simulink library "ModelsLibrary"  (R2017b)
settings: Solver=VariableStepAuto  StartTime=0.0  StopTime=10.0  RelTol=1e-3
libraries: sharedutil x3, simulink x2, ModelsLibrary x2
settings Model: Creator=AHKh  LastModifiedBy=AHKh
settings CodeAppCC: StateflowObjectComments=on

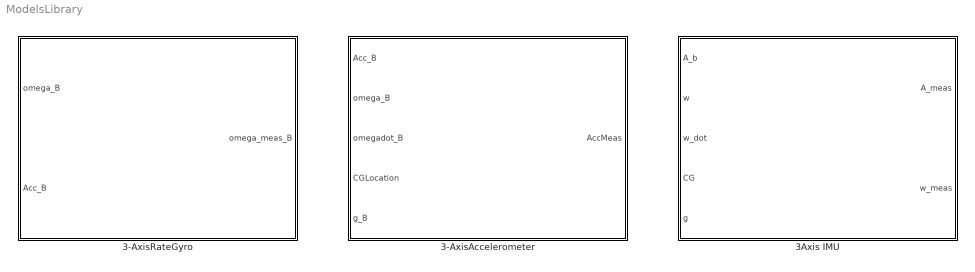
== system ModelsLibrary ==
  3-AxisAccelerometer : Subsystem  mask{units=Metric (MKS), SensorLoc=[0; 0; 0], gtype=off, dtype_a=on, w_a=190, z_a=0.707, SFCC=eye(3), SensorBias=[0; 0; 0], Ts=0.001, AccNoiseCheck=on, NoiseSeeds=[23093; 23094; 23095], NoisePower=[0.001; 0.001; 0.001], satUpper=[inf; inf; inf], satLower=[-inf; -inf; -inf]}
      mask prompts: units "Unit"; SensorLoc "Accelerometer Location"; gtype "Subtracting Gravity"; dtype_a "Considering 2nd-Order Dynamics"; w_a "Natural Frequency (rad/s)"; z_a "Damping Ratio"; SFCC "Scale Factor and Cross-Coupling"; SensorBias "Measurment Bias"; Ts "Update Rate (sec)"; AccNoiseCheck "Considering Noise"; NoiseSeeds "Noise Seeds"; NoisePower "Noise Power"; satUpper "Output Upper Limits"; satLower "Output Lower Limits"
      mask TypeOptions units: Metric (MKS)
      mask DialogControl DescGroupVar Prompt: Three-Axis Accelerometer
      mask DialogControl DescTextVar Prompt: Implements a three-axis accelerometer
      mask DialogControl Container4 Prompt: Main
      mask DialogControl units Tooltip: Metric System of Units
      mask DialogControl Container5 Prompt: Noise Characteristics
      mask Display:
      | port_label('input',1,'[Acc]^{B}_B (m/s^2)','texmode','on');
      | port_label('input',2,'[\omega]^B_B (rad/s)','texmode','on');
      | port_label('input',3,'[d\omega/dt]^B_B (rad/s^2)','texmode','on');
      | port_label('input',4,'[CG]^B_B (m)','texmode','on');
      | port_label('input',5,'[g]^B_B (m/s^2)','texmode','on');
      | port_label('output',1,'[Acc_{meas}]^{B}_B (m/s^2)','texmode','on');
  3-AxisRateGyro : Subsystem  mask(Three-Axis Rate Gyroscope){dtype_g=on, w_g=190, z_g=0.707, SFCC=eye(3), SensorBias=[0; 0; 0], gSensitivity=[0; 0; 0], Ts=0.001, GyroNoiseCheck=on, NoiseSeeds=[23093; 23094; 23095], NoisePower=[0.0001; 0.0001; 0.0001], satUpper=[inf; inf; inf], satLower=[-inf; -inf; -inf]}
      mask prompts: dtype_g "Considering 2nd-Order Dynamics"; w_g "Natural Frequency (rad/s)"; z_g "Damping Ratio"; SFCC "Scale Factors and Cross-Coupling"; SensorBias "Measurment Bias"; gSensitivity "G-Sensitive Bias"; Ts "Update Rate (sec)"; GyroNoiseCheck "Considering Noise"; NoiseSeeds "Noise Seeds"; NoisePower "Noise Power"; satUpper "Output Upper Bound"; satLower "Output Lower Bound"
      mask DialogControl DescGroupVar Prompt: Three-Axis Gyroscope
      mask DialogControl DescTextVar Prompt: Implements a three-axis gyroscope.
      mask DialogControl Container4 Prompt: Main
      mask DialogControl Container5 Prompt: Noise Characteristics
      mask Display:
      | port_label('input',1,'[\omega]^B_B (rad/s)','texmode','on');
      | port_label('input',2,'[Acc]^{B}_B (m/s^2)','texmode','on');
      | port_label('output',1,'[\omega_{meas}]^{B}_B (rad/s)','texmode','on');
  3Axis IMU : Subsystem  mask{units=Metric (MKS), IMULocation=[0; 0; 0], Ts=0.001, AccSubtractGravity=off, dtype_a=on, AccNaturalFrequency=190, AccDampingRatio=0.707, AccSFCC=eye(3), AccMeasurmentBias=[0; 0; 0], AccMeasUpperLimit=[inf; inf; inf], AccMeasLowerLimit=[-inf; -inf; -inf], AccNoiseCheck=on, AccNoiseSeeds=[23093; 23094; 23095], AccNoisePower=[0.0001; 0.0001; 0.0001], dtype_g=on, GyroNaturalFrequency=190, GyroDampingRatio=0.707, GyroSFCC=eye(3), GyroMeasurmentBias=[0; 0; 0], GyroGSensitiveBias=[0; 0; 0], GyroMeasUpperLimit=[inf; inf; inf], GyroMeasLowerLimit=[-inf; -inf; -inf], GyroNoiseCheck=on, GyroNoiseSeeds=[23093; 23094; 23095], GyroNoisePower=[0.0001; 0.0001; 0.0001]}
      mask prompts: IMULocation "IMU Location (m)"; Ts "Update Rate (sec)"; AccSubtractGravity "Subtracting Gravity"; dtype_a "Considering 2nd-Order Dynamics"; AccNaturalFrequency "Natural Frequency (rad/s)"; AccDampingRatio "Damping Ratio"; AccSFCC "Scale Factor and Cross Coupling"; AccMeasurmentBias "Measurment Bias"; AccMeasUpperLimit "Measurment Upper Limit"; AccMeasLowerLimit "Measurment Lower Limit"; AccNoiseCheck "Considering Noise"; AccNoiseSeeds "Noise Seeds"; AccNoisePower "Noise Power"; dtype_g "Considering 2nd-Order Dynamics"; GyroNaturalFrequency "Natural Frequency (rad/s)"; GyroDampingRatio "Damping Ratio"; GyroSFCC "Scale Factor and Cross Coupling"; GyroMeasurmentBias "Measurment Bias"; GyroGSensitiveBias "G-Sensitive Bias"; GyroMeasUpperLimit "Measurment Upper Limit"; GyroMeasLowerLimit "Measurment Lower Limit"; GyroNoiseCheck "Considering Noise"; GyroNoiseSeeds "Noise Seeds"; GyroNoisePower "Noise Power"
      mask init:
      | a1 = get(gcbh,'AccSubtractGravity');
      | a2 = get(gcbh,'dtype_a');
      | a3 = get(gcbh,'AccNoiseCheck');
      | a4 = get(gcbh,'dtype_g');
      | a5 = get(gcbh,'GyroNoiseCheck');
      | Acc = getSimulinkBlockHandle([gcb '/3-AxisAccelerometer']);
      | Gyro = getSimulinkBlockHandle([gcb '/3-AxisRateGyro']);
      | set(Acc,'gtype',a1);
      | set(Acc,'dtype_a',a2);
      | set(Acc,'AccNoiseCheck',a3);
      | set(Gyro,'dtype_g',a4);
      | set(Gyro,'GyroNoiseCheck',a5);
      mask TypeOptions units: Metric (MKS)
      mask DialogControl DescGroupVar Prompt: 3-Axis IMU
      mask DialogControl DescTextVar Prompt: Implements 3-axis Inertial Measurment Unit (IMU)
      mask DialogControl Container4 Prompt: Main
      mask DialogControl Container9 Prompt: Accelerometer
      mask DialogControl Container11 Prompt: Accelerometer General
      mask DialogControl Container14 Prompt: Accelerometer Noise
      mask DialogControl Container5 Prompt: Gyroscope
      mask DialogControl Container7 Prompt: Gyroscope General
      mask DialogControl Container8 Prompt: Gyroscope Noise
      mask Display:
      | port_label('input',1,'[Acc]^{B}_B (m/s^2)','texmode','on');
      | port_label('input',2,'[\omega]^B_B (rad/s)','texmode','on');
      | port_label('input',3,'[d\omega/dt]^B_B (rad/s^2)','texmode','on');
      | port_label('input',4,'[CG]^B_B (m)','texmode','on');
      | port_label('input',5,'[g]^B_B (m/s^2)','texmode','on');
      | port_label('output',1,'[Acc_{meas}]^{B}_B (m/s^2)','texmode','on');
      | port_label('output',2,'[\omega_{meas}]^{B}_B (rad/s)','texmode','on');

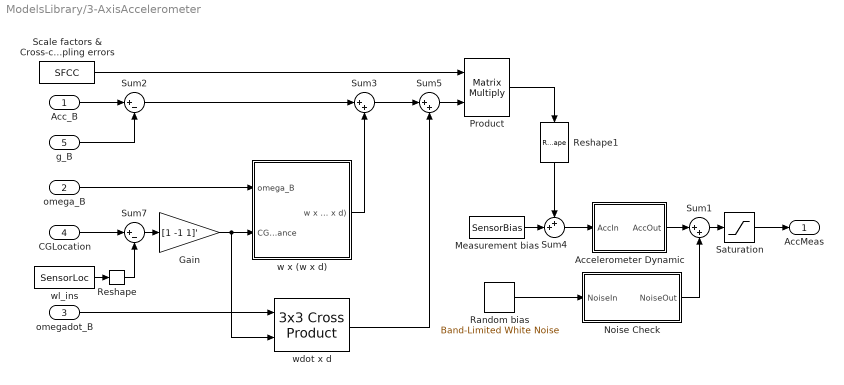
== system ModelsLibrary/3-AxisAccelerometer ==
  Acc_B : Inport  Unit=m/s^2  PortDimensions=[3,1]
  omega_B : Inport  Port=2  Unit=rad/s  PortDimensions=[3,1]
  omegadot_B : Inport  Port=3  Unit=rad/s^2  PortDimensions=[3,1]
  CGLocation : Inport  Port=4  Unit=m  PortDimensions=[3,1]
  g_B : Inport  Port=5  Unit=m/s^2  PortDimensions=[3,1]
  Accelerometer Dynamic : Subsystem
  Gain : Gain  Gain=[1 -1 1]'  SaturateOnIntegerOverflow=on  OutDataTypeStr=Inherit: Same as input  ParamDataTypeStr=Inherit: Same as input
  Measurement bias : Constant  Value=SensorBias
  Noise Check : Subsystem
  Product : Product  Multiplication=Matrix(*)  SaturateOnIntegerOverflow=on  OutDataTypeStr=Inherit: Same as first input
  Random bias : simulink/Sources/Band-Limited White Noise  Cov=NoisePower  Ts=Ts  seed=NoiseSeeds
  Reshape : Reshape  OutputDimensionality=Column vector (2-D)
  Reshape1 : Reshape
  Saturation : Saturate  UpperLimit=satUpper  LowerLimit=satLower
  Scale factors & Cross-coupling errors : Constant  Value=SFCC
  Sum1 : Sum  Inputs=|++  SaturateOnIntegerOverflow=on
  Sum2 : Sum  Inputs=|+-
  Sum3 : Sum  Inputs=|++
  Sum4 : Sum  Inputs=++|  SaturateOnIntegerOverflow=on
  Sum5 : Sum  Inputs=|++
  Sum7 : Sum  Inputs=|+-  SaturateOnIntegerOverflow=on
  w x (w x d) : Subsystem
  wdot x d : sharedutil/3x3 Cross Product
      settings: SourceProductBaseCode=AE
  wl_ins : Constant  Value=SensorLoc
  AccMeas : Outport  Unit=m/s^2  PortDimensions=[3,1]
  wires:
  Gain/1 -> w x (w x d)/2(CGAccdistance), wdot x d/2
  Sum4/1 -> Accelerometer Dynamic/1(AccIn)
  omegadot_B/1 -> wdot x d/1
  omega_B/1 -> w x (w x d)/1(omega_B)
  Scale factors & Cross-coupling errors/1 -> Product/1
  Measurement bias/1 -> Sum4/2
  Sum7/1 -> Gain/1
  wdot x d/1 -> Sum5/2
  CGLocation/1 -> Sum7/1
  Accelerometer Dynamic/1("AccOut ") -> Sum1/1
  Saturation/1 -> AccMeas/1
  Product/1 -> Reshape1/1
  Sum1/1 -> Saturation/1
  Random bias/1 -> Noise Check/1(NoiseIn)
  Reshape1/1 -> Sum4/1
  Sum5/1 -> Product/2
  Acc_B/1 -> Sum2/1
  g_B/1 -> Sum2/2
  Sum2/1 -> Sum3/1
  w x (w x d)/1(w x ( w x d)) -> Sum3/2
  Sum3/1 -> Sum5/1
  wl_ins/1 -> Reshape/1
  Reshape/1 -> Sum7/2
  Noise Check/1("NoiseOut ") -> Sum1/2

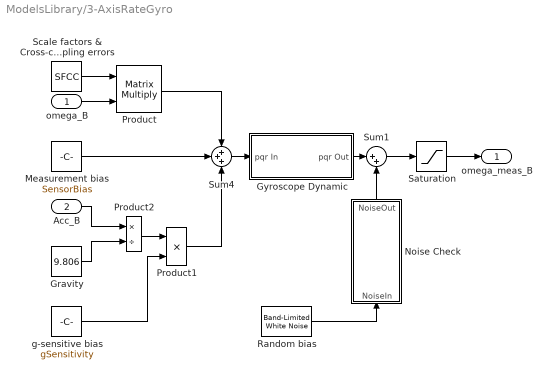
== system ModelsLibrary/3-AxisRateGyro ==
  omega_B : Inport  Unit=rad/s  PortDimensions=3
  Acc_B : Inport  Port=2  Unit=m/s^2  PortDimensions=3
  Gravity : Constant  Value=9.806
  Gyroscope Dynamic : Subsystem
  Measurement bias : Constant  Value=SensorBias
  Noise Check : Subsystem
  Product : Product  Multiplication=Matrix(*)  SaturateOnIntegerOverflow=on  OutDataTypeStr=Inherit: Same as first input
  Product1 : Product  SaturateOnIntegerOverflow=on  OutDataTypeStr=Inherit: Same as first input
  Product2 : Product  Inputs=*/  SaturateOnIntegerOverflow=on  OutDataTypeStr=Inherit: Same as first input
  Random bias : simulink/Sources/Band-Limited White Noise  Cov=NoisePower  Ts=Ts  seed=NoiseSeeds
  Saturation : Saturate  UpperLimit=satUpper  LowerLimit=satLower
  "Scale factors & Cross-coupling errors " : Constant  Value=SFCC
  Sum1 : Sum  Inputs=|++  SaturateOnIntegerOverflow=on
  Sum4 : Sum  Inputs=+++  SaturateOnIntegerOverflow=on
  g-sensitive bias : Constant  Value=gSensitivity
  omega_meas_B : Outport  Unit=rad/s
  wires:
  Product/1 -> Sum4/1
  Gyroscope Dynamic/1(pqr Out) -> Sum1/1
  Acc_B/1 -> Product2/1
  Product2/1 -> Product1/1
  Sum1/1 -> Saturation/1
  omega_B/1 -> Product/2
  Random bias/1 -> Noise Check/1(NoiseIn)
  Saturation/1 -> omega_meas_B/1
  Measurement bias/1 -> Sum4/2
  "Scale factors & Cross-coupling errors "/1 -> Product/1
  Sum4/1 -> Gyroscope Dynamic/1(pqr In)
  g-sensitive bias/1 -> Product1/2
  Product1/1 -> Sum4/3
  Gravity/1 -> Product2/2
  Noise Check/1("NoiseOut ") -> Sum1/2

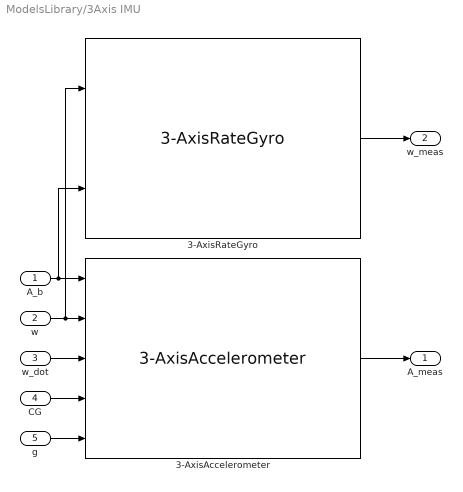
== system ModelsLibrary/3Axis IMU ==
  A_b : Inport  Unit=m/s^2  PortDimensions=[3,1]
  w : Inport  Port=2  Unit=rad/s  PortDimensions=[3,1]
  w_dot : Inport  Port=3  Unit=rad/s^2  PortDimensions=[3,1]
  CG : Inport  Port=4  Unit=m  PortDimensions=[3,1]
  g : Inport  Port=5  Unit=m/s^2  PortDimensions=[3,1]
  3-AxisAccelerometer : ModelsLibrary/3-AxisAccelerometer  units=Metric (MKS)  SensorLoc=IMULocation  gtype=off  dtype_a=on  w_a=AccNaturalFrequency  z_a=AccDampingRatio  SFCC=AccSFCC  SensorBias=AccMeasurmentBias  Ts=Ts  AccNoiseCheck=on  NoiseSeeds=AccNoiseSeeds  NoisePower=AccNoisePower  satUpper=AccMeasUpperLimit  satLower=AccMeasLowerLimit
  3-AxisRateGyro : ModelsLibrary/3-AxisRateGyro  dtype_g=on  w_g=GyroNaturalFrequency  z_g=GyroDampingRatio  SFCC=GyroSFCC  SensorBias=GyroMeasurmentBias  gSensitivity=GyroGSensitiveBias  Ts=Ts  GyroNoiseCheck=on  NoiseSeeds=GyroNoiseSeeds  NoisePower=GyroNoisePower  satUpper=GyroMeasUpperLimit  satLower=GyroMeasLowerLimit
  A_meas : Outport  Unit=m/s^2  PortDimensions=[3,1]
  w_meas : Outport  Port=2  Unit=rad/s  PortDimensions=[3,1]
  wires:
  3-AxisRateGyro/1 -> w_meas/1
  w/1 -> 3-AxisRateGyro/1, 3-AxisAccelerometer/2
  A_b/1 -> 3-AxisRateGyro/2, 3-AxisAccelerometer/1
  3-AxisAccelerometer/1 -> A_meas/1
  w_dot/1 -> 3-AxisAccelerometer/3
  CG/1 -> 3-AxisAccelerometer/4
  g/1 -> 3-AxisAccelerometer/5

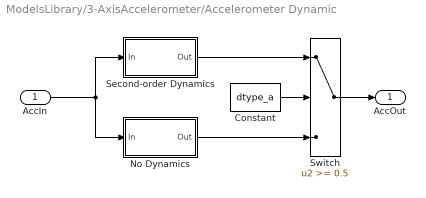
== system ModelsLibrary/3-AxisAccelerometer/Accelerometer Dynamic ==
  AccIn : Inport
  Constant : Constant  Value=dtype_a
  No Dynamics : Subsystem
  Second-order Dynamics : Subsystem
  Switch : Switch  Threshold=0.5
  "AccOut " : Outport
  wires:
  Constant/1 -> Switch/2
  Switch/1 -> "AccOut "/1
  Second-order Dynamics/1("Out ") -> Switch/1
  AccIn/1 -> No Dynamics/1(In), Second-order Dynamics/1(In)
  No Dynamics/1("Out ") -> Switch/3

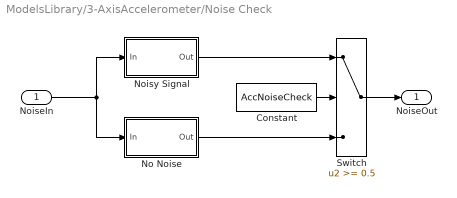
== system ModelsLibrary/3-AxisAccelerometer/Noise Check ==
  NoiseIn : Inport
  Constant : Constant  Value=AccNoiseCheck
  No Noise : Subsystem
  Noisy Signal : Subsystem
  Switch : Switch  Threshold=0.5
  "NoiseOut " : Outport
  wires:
  NoiseIn/1 -> No Noise/1(In), Noisy Signal/1(In)
  No Noise/1("Out ") -> Switch/3
  Noisy Signal/1("Out ") -> Switch/1
  Switch/1 -> "NoiseOut "/1
  Constant/1 -> Switch/2

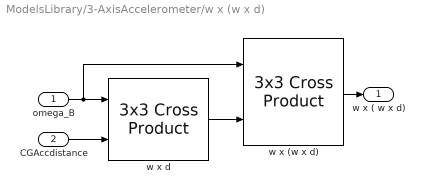
== system ModelsLibrary/3-AxisAccelerometer/w x (w x d) ==
  omega_B : Inport  PortDimensions=[3,1]
  CGAccdistance : Inport  Port=2  PortDimensions=[3,1]
  w x (w x d) : sharedutil/3x3 Cross Product
      settings: SourceProductBaseCode=AE
  w x d : sharedutil/3x3 Cross Product
      settings: SourceProductBaseCode=AE
  w x ( w x d) : Outport  PortDimensions=[3,1]
  wires:
  w x d/1 -> w x (w x d)/2
  CGAccdistance/1 -> w x d/2
  omega_B/1 -> w x (w x d)/1, w x d/1
  w x (w x d)/1 -> w x ( w x d)/1

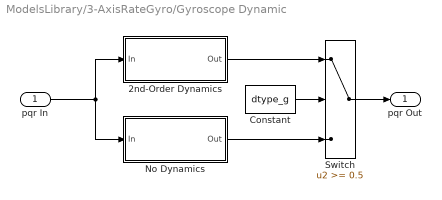
== system ModelsLibrary/3-AxisRateGyro/Gyroscope Dynamic ==
  pqr In : Inport  PortDimensions=[3,1]
  2nd-Order Dynamics : Subsystem
  Constant : Constant  Value=dtype_g
  No Dynamics : Subsystem
  Switch : Switch  Threshold=0.5
  pqr Out : Outport  SampleTime=[3,1]
  wires:
  pqr In/1 -> No Dynamics/1(In), 2nd-Order Dynamics/1(In)
  Constant/1 -> Switch/2
  No Dynamics/1(Out) -> Switch/3
  2nd-Order Dynamics/1(Out) -> Switch/1
  Switch/1 -> pqr Out/1

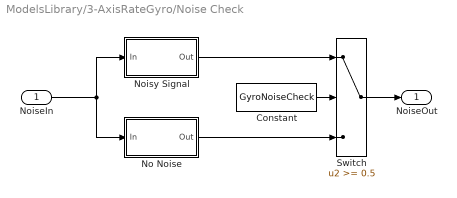
== system ModelsLibrary/3-AxisRateGyro/Noise Check ==
  NoiseIn : Inport
  Constant : Constant  Value=GyroNoiseCheck
  No Noise : Subsystem
  Noisy Signal : Subsystem
  Switch : Switch  Threshold=0.5
  "NoiseOut " : Outport
  wires:
  Constant/1 -> Switch/2
  Switch/1 -> "NoiseOut "/1
  Noisy Signal/1("Out ") -> Switch/1
  No Noise/1("Out ") -> Switch/3
  NoiseIn/1 -> Noisy Signal/1(In), No Noise/1(In)

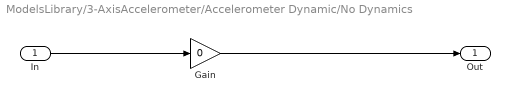
== system ModelsLibrary/3-AxisAccelerometer/Accelerometer Dynamic/No Dynamics ==
  In : Inport
  Gain : Gain  Gain=0
  "Out " : Outport
  wires:
  In/1 -> Gain/1
  Gain/1 -> "Out "/1

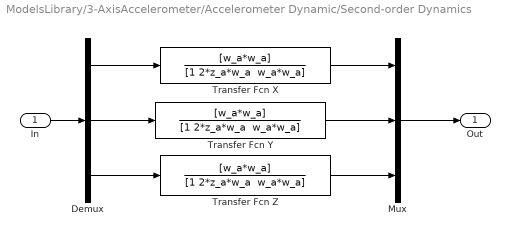
== system ModelsLibrary/3-AxisAccelerometer/Accelerometer Dynamic/Second-order Dynamics ==
  In : Inport
  Demux : Demux  Outputs=3
  Mux : Mux  Inputs=3
  Transfer Fcn X : TransferFcn  Numerator=[w_a*w_a]  Denominator="[1 2*z_a*w_a  w_a*w_a]"
  Transfer Fcn Y : TransferFcn  Numerator=[w_a*w_a]  Denominator="[1 2*z_a*w_a  w_a*w_a]"
  Transfer Fcn Z : TransferFcn  Numerator=[w_a*w_a]  Denominator="[1 2*z_a*w_a  w_a*w_a]"
  "Out " : Outport
  wires:
  Transfer Fcn Y/1 -> Mux/2
  In/1 -> Demux/1
  Demux/1 -> Transfer Fcn X/1
  Transfer Fcn Z/1 -> Mux/3
  Demux/2 -> Transfer Fcn Y/1
  Demux/3 -> Transfer Fcn Z/1
  Mux/1 -> "Out "/1
  Transfer Fcn X/1 -> Mux/1

== system ModelsLibrary/3-AxisAccelerometer/Noise Check/No Noise ==
  In : Inport
  Gain : Gain  Gain=0
  "Out " : Outport
  wires:
  In/1 -> Gain/1
  Gain/1 -> "Out "/1

== system ModelsLibrary/3-AxisAccelerometer/Noise Check/Noisy Signal ==
  In : Inport
  "Out " : Outport
  wires:
  In/1 -> "Out "/1

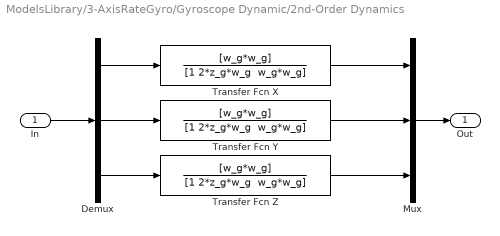
== system ModelsLibrary/3-AxisRateGyro/Gyroscope Dynamic/2nd-Order Dynamics ==
  In : Inport  PortDimensions=[3,1]
  Demux : Demux  Outputs=3
  Mux : Mux  Inputs=3
  Transfer Fcn X : TransferFcn  Numerator=[w_g*w_g]  Denominator="[1 2*z_g*w_g  w_g*w_g]"
  Transfer Fcn Y : TransferFcn  Numerator=[w_g*w_g]  Denominator="[1 2*z_g*w_g  w_g*w_g]"
  Transfer Fcn Z : TransferFcn  Numerator=[w_g*w_g]  Denominator="[1 2*z_g*w_g  w_g*w_g]"
  Out : Outport  PortDimensions=[3,1]
  wires:
  In/1 -> Demux/1
  Demux/3 -> Transfer Fcn Z/1
  Demux/2 -> Transfer Fcn Y/1
  Mux/1 -> Out/1
  Transfer Fcn Y/1 -> Mux/2
  Transfer Fcn X/1 -> Mux/1
  Demux/1 -> Transfer Fcn X/1
  Transfer Fcn Z/1 -> Mux/3

== system ModelsLibrary/3-AxisRateGyro/Gyroscope Dynamic/No Dynamics ==
  In : Inport  PortDimensions=[3,1]
  Out : Outport  PortDimensions=[3,1]
  wires:
  In/1 -> Out/1

== system ModelsLibrary/3-AxisRateGyro/Noise Check/No Noise ==
  In : Inport
  Gain : Gain  Gain=0
  "Out " : Outport
  wires:
  Gain/1 -> "Out "/1
  In/1 -> Gain/1

== system ModelsLibrary/3-AxisRateGyro/Noise Check/Noisy Signal ==
  In : Inport
  "Out " : Outport
  wires:
  In/1 -> "Out "/1
